simulink model "ModelloSospensioneSubsystemPID"  (R2017a)
settings: Solver=FixedStepAuto  StartTime=0.0  StopTime=10  FixedStep=0.01  RelTol=1e-3
undefined symbols (not defined in the file): c1, c2, k1, k2, m1, m2
libraries: simulink x1
settings Model: Creator=Karimo  LastModifiedBy=Karimo

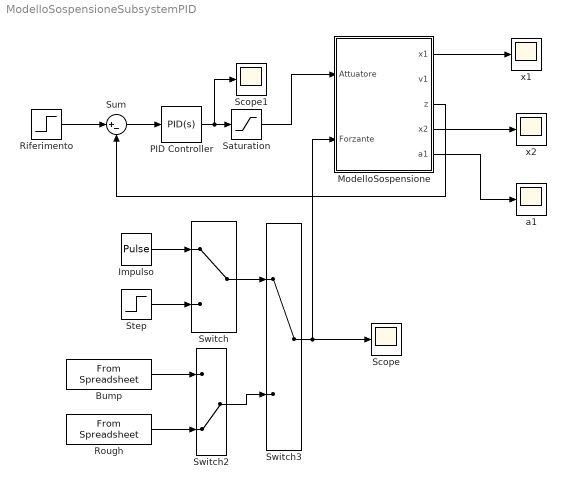
== system ModelloSospensioneSubsystemPID ==
  Bump : FromSpreadsheet  FileName=C:\Users\Karimo\Desktop\UNITS\Meccanica delle vibrazioni\Bump.xlsx  SheetName=Foglio1
  Impulso : DiscretePulseGenerator  PulseType=Time based  Amplitude=0.1  Period=10  PulseWidth=0.1  PhaseDelay=1
  ModelloSospensione : Subsystem
  PID Controller : simulink/Continuous/PID Controller  Controller=PID  TimeDomain=Continuous-time  SampleTime=-1  IntegratorMethod=Forward Euler  FilterMethod=Forward Euler  Form=Parallel  UseFilter=on  ControllerParametersSource=internal  P=500  I=10000  D=900  N=100  InitialConditionSource=internal  InitialConditionForIntegrator=0  InitialConditionForFilter=0  ExternalReset=none  LimitOutput=off  UpperSaturationLimit=inf  LowerSaturationLimit=-inf  LinearizeAsGain=on  AntiWindupMode=none  Kb=1  TrackingMode=off  Kt=1  PParamMin=[]  PParamMax=[]  IParamMin=[]  IParamMax=[]  DParamMin=[]  DParamMax=[]  NParamMin=[]  NParamMax=[]  KbParamMin=[]  KbParamMax=[]  KtParamMin=[]  KtParamMax=[]  POutMin=[]  POutMax=[]  IOutMin=[]  IOutMax=[]  DOutMin=[]  DOutMax=[]  NOutMin=[]  NOutMax=[]  KbOutMin=[]  KbOutMax=[]  KtOutMin=[]  KtOutMax=[]  IntegratorOutMin=[]  IntegratorOutMax=[]  FilterOutMin=[]  FilterOutMax=[]  SumOutMin=[]  SumOutMax=[]  SumI1OutMin=[]  SumI1OutMax=[]  SumI2OutMin=[]  SumI2OutMax=[]  SumI3OutMin=[]  SumI3OutMax=[]  SumDOutMin=[]  SumDOutMax=[]  SaturationOutMin=[]  SaturationOutMax=[]  IntegratorContinuousStateAttributes=''  IntegratorStateMustResolveToSignalObject=off  IntegratorRTWStateStorageClass=Auto  FilterContinuousStateAttributes=''  FilterStateMustResolveToSignalObject=off  FilterRTWStateStorageClass=Auto  DifferentiatorICPrevScaledInput=0  DifferentiatorOutMin=[]  DifferentiatorOutMax=[]  InitialConditionSetting=State (most efficient)
  Riferimento : Step  Time=0  After=0  SampleTime=0
  Rough : FromSpreadsheet  FileName=C:\Users\Karimo\Desktop\UNITS\Meccanica delle vibrazioni\Rough.xlsx  SheetName=Foglio1
  Saturation : Saturate  UpperLimit=1500  LowerLimit=-1500
  Scope : Scope
  Scope1 : Scope
  Step : Step  Time=5  After=0.1  SampleTime=0
  Sum : Sum  Inputs=|+-
  Switch : ManualSwitch
  Switch2 : ManualSwitch  CurrentSetting=0
  Switch3 : ManualSwitch
  a1 : Scope
  x1 : Scope
  x2 : Scope
  wires:
  PID Controller/1 -> Scope1/1, Saturation/1
  Riferimento/1 -> Sum/1
  Sum/1 -> PID Controller/1
  ModelloSospensione/3(z) -> Sum/2
  ModelloSospensione/1(x1) -> x1/1
  Saturation/1 -> ModelloSospensione/1(Attuatore)
  ModelloSospensione/4(x2) -> x2/1
  ModelloSospensione/5(a1) -> a1/1
  Impulso/1 -> Switch/1
  Switch3/1 -> ModelloSospensione/2(Forzante), Scope/1
  Step/1 -> Switch/2
  Bump/1 -> Switch2/1
  Rough/1 -> Switch2/2
  Switch/1 -> Switch3/1
  Switch2/1 -> Switch3/2

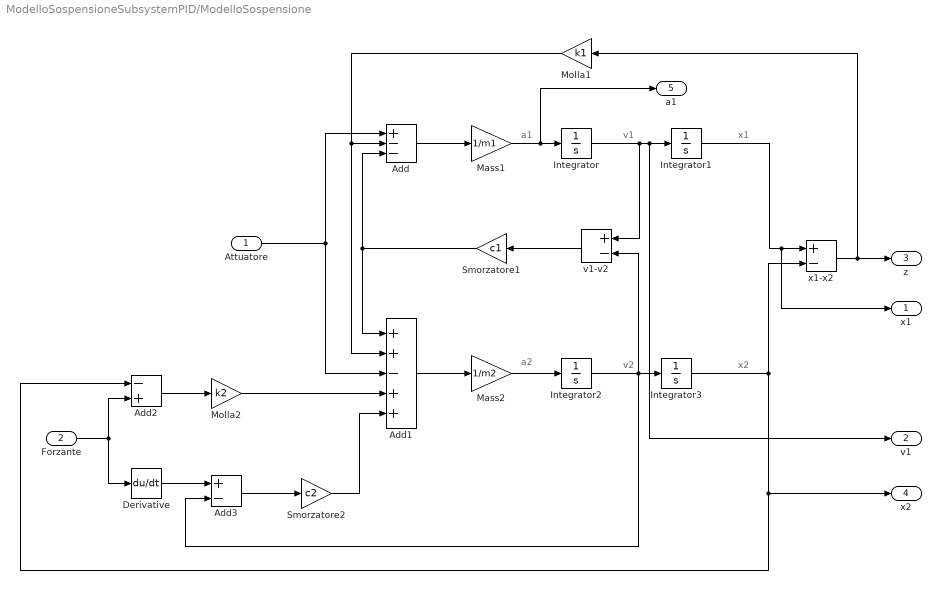
== system ModelloSospensioneSubsystemPID/ModelloSospensione ==
  note: a2
  note: x1
  note: v1
  note: a1
  note: v2
  note: x2
  Attuatore : Inport
  Forzante : Inport  Port=2
  Add : Sum  Inputs=+--
  Add1 : Sum  Inputs=++-++
  Add2 : Sum  Inputs=-+
  Add3 : Sum  Inputs=+-
  Derivative : Derivative
  Integrator{,1..3} (4 alike) : Integrator
  Mass1 : Gain  Gain=1/m1
  Mass2 : Gain  Gain=1/m2
  Molla1 : Gain  Gain=k1
  Molla2 : Gain  Gain=k2
  Smorzatore1 : Gain  Gain=c1
  Smorzatore2 : Gain  Gain=c2
  v1-v2 : Sum  Inputs=+-
  x1-x2 : Sum  Inputs=+-
  x1 : Outport
  v1 : Outport  Port=2
  z : Outport  Port=3
  x2 : Outport  Port=4
  a1 : Outport  Port=5
  wires:
  Add3/1 -> Smorzatore2/1
  x1-x2/1 -> z/1, Molla1/1
  Molla1/1 -> Add1/2, Add/2
  Smorzatore2/1 -> Add1/5
  Add2/1 -> Molla2/1
  Molla2/1 -> Add1/4
  Attuatore/1 -> Add/1, Add1/3
  Add/1 -> Mass1/1
  Mass2/1 -> Integrator2/1
  Forzante/1 -> Add2/2, Derivative/1
  Integrator3/1 -> x2/1, Add2/1, x1-x2/2
  Integrator2/1 -> Add3/2, v1-v2/2, Integrator3/1
  Mass1/1 -> a1/1, Integrator/1
  Smorzatore1/1 -> Add1/1, Add/3
  Derivative/1 -> Add3/1
  Add1/1 -> Mass2/1
  v1-v2/1 -> Smorzatore1/1
  Integrator1/1 -> x1-x2/1, x1/1
  Integrator/1 -> v1-v2/1, v1/1, Integrator1/1
